simulink model "drivelinemodel"  (R2017b)
settings: Solver=VariableStepAuto  StartTime=0.0  StopTime=17.0  MaxStep=0.001  RelTol=1e-3
values from neighbouring files (symbols this model uses):
  A = [-ds/(Jf*r^2) ds/(Jf*r) -cs/(Jf*r) ... (first row only)    [driveline.m]
  B1 = [B H]    [driveline.m]
  C = eye(3)    [driveline.m]
  D = zeros(3,2)    [driveline.m]
  x0 = [120 2 0]'    [driveline.m]
settings Model: Creator=jofr  LastModifiedBy=jofr

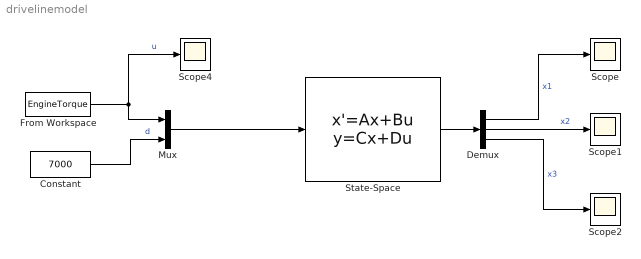
== system drivelinemodel ==
  Constant : Constant  Value=7000
  Demux : Demux  Outputs=3
  From Workspace : FromWorkspace  VariableName=EngineTorque  SampleTime=0
  Mux : Mux  Inputs=2
  Scope{,1..2,4} (4 alike) : Scope
  State-Space : StateSpace  A=A  B=B1  C=C  D=D  InitialCondition=x0
  wires:
  State-Space/1 -> Demux/1
  Demux/1 -> Scope/1  "x1"
  Demux/2 -> Scope1/1  "x2"
  Demux/3 -> Scope2/1  "x3"
  Mux/1 -> State-Space/1
  Constant/1 -> Mux/2  "d"
  From Workspace/1 -> Scope4/1, Mux/1  "u"
